simulink model "simulation"  (R2023b)
settings: Solver=VariableStepAuto  StartTime=0.0  StopTime=10.0  RelTol=1e-3
InitFcn:
  | param = plant_param();
  | sysc = plant_sysc(param);
undefined symbols (not defined in the file or in its folder): x0
settings Model: Creator=block  LastModifiedBy=block

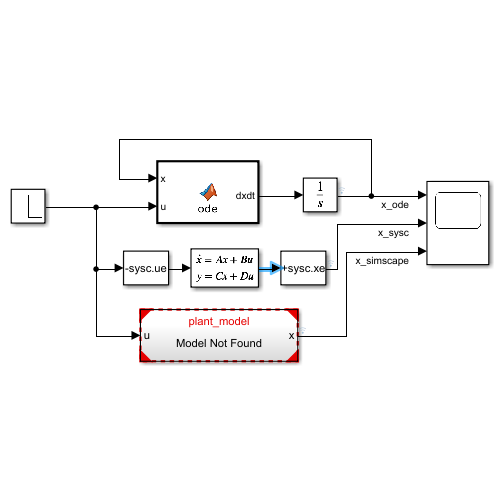
[thumbnail: Simulink's stored preview of the top-level diagram]
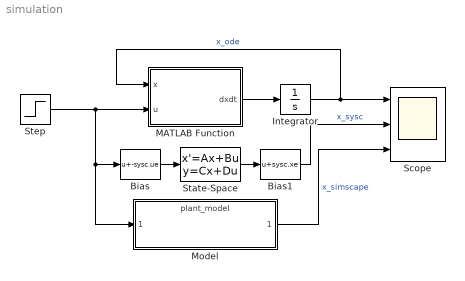
== system simulation ==
  Bias : Bias  Bias=-sysc.ue  SaturateOnIntegerOverflow=off
  Bias1 : Bias  Bias=sysc.xe  SaturateOnIntegerOverflow=off
  Integrator : Integrator  InitialCondition=x0
  MATLAB Function : MATLAB Function  TreatAsAtomicUnit=on
  Model : ModelReference  ModelNameDialog=plant_model  SimulationMode=Normal  ModelReferenceVersion=1.4
  Scope : Scope  NumInputPorts=3
  State-Space : StateSpace  A=sysc.A  B=sysc.B  C=sysc.C  D=sysc.D  InitialCondition=x0-sysc.xe
  Step : Step  Time=0.01  Before=100  After=0  SampleTime=0
  wires:
  Bias1/1 -> Scope/2  "x_sysc"
  MATLAB Function/1(dxdt) -> Integrator/1
  Integrator/1 -> Scope/1, MATLAB Function/1(x)  "x_ode"
  Step/1 -> MATLAB Function/2(u), Model/1, Bias/1
  Model/1 -> Scope/3  "x_simscape"
  Bias/1 -> State-Space/1
  State-Space/1 -> Bias1/1

== matlab function simulation/MATLAB Function ==
  data: x input; u input; dxdt output; param parameter
function dxdt = ode(x,u,param)
    dxdt = plant_ode(0,x,u,param);
end
